simulink model "blocos"  (R2023b)
settings: Solver=VariableStepAuto  StartTime=0.0  StopTime=0.3  RelTol=1e-3
undefined symbols (not defined in the file or in its folder): b, f_final, f_inicial, k, m, t_inicial
settings Model: Creator=thiag  LastModifiedBy=thiag

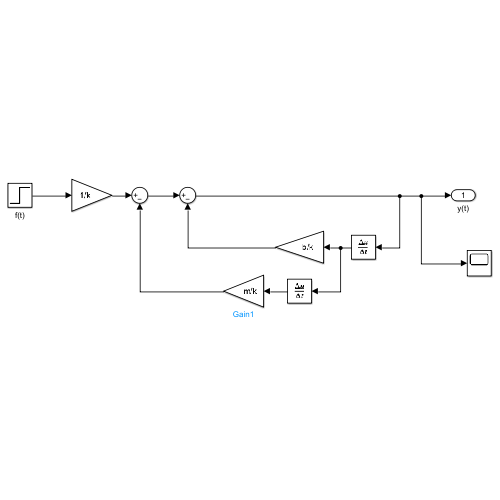
[thumbnail: Simulink's stored preview of the top-level diagram]
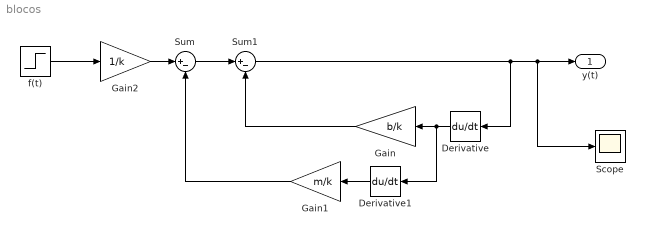
== system blocos ==
  Derivative : Derivative
  Derivative1 : Derivative
  Gain : Gain  Gain=b/k
  Gain1 : Gain  Gain=m/k
  Gain2 : Gain  Gain=1/k
  Scope : Scope
  Sum : Sum  Inputs=|+-
  Sum1 : Sum  Inputs=|+-
  f(t) : Step  Time=t_inicial  Before=f_inicial  After=f_final  SampleTime=0
  y(t) : Outport
  wires:
  Derivative/1 -> Derivative1/1, Gain/1
  Derivative1/1 -> Gain1/1
  Sum1/1 -> Derivative/1, Scope/1, y(t)/1
  Gain/1 -> Sum1/2
  Gain1/1 -> Sum/2
  Sum/1 -> Sum1/1
  Gain2/1 -> Sum/1
  f(t)/1 -> Gain2/1
